simulink model "sim_suspension"  (R2024a)
settings: Solver=ode45  StartTime=0.0  StopTime=3  MaxStep=1e-3  RelTol=1e-3
model workspace (MAT data in the model file):
  road_excitation = 20
undefined symbols (not defined in the file): k, m, r, road_excitation_amplitude, road_excitation_omega, v0, x0
settings Model: Creator=ArrigonDell  LastModifiedBy=Bocchio
settings SolverCC: AlgebraicLoopSolver=TrustRegion
settings DataIOCC: SaveOutput=off  SaveTime=off  ReturnWorkspaceOutputs=off
settings DebuggingCC: UnconnectedInputMsg=warning  UnconnectedOutputMsg=warning  UnconnectedLineMsg=warning  ArithmeticOperatorsInVariantConditions=warning
settings ModelReferenceCC: EnableRefExpFcnMdlSchedulingChecks=on
settings SFSimCC: SimUseLocalCustomCode=off  CustomCodeUndefinedFunction=UseInterfaceOnly
settings RTWCC: RTWUseLocalCustomCode=off  GPUComputeCapability=3.5  DLArmComputeVersion=19.05

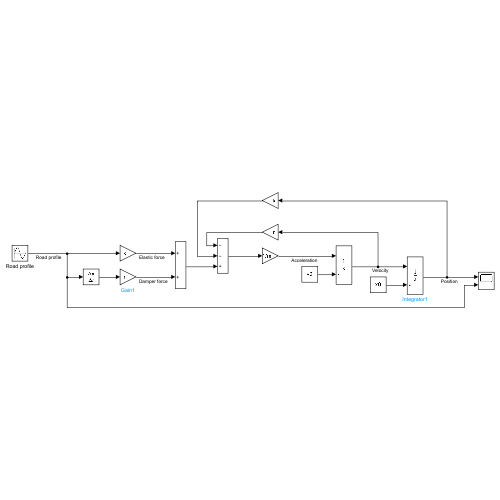
[thumbnail: Simulink's stored preview of the top-level diagram]
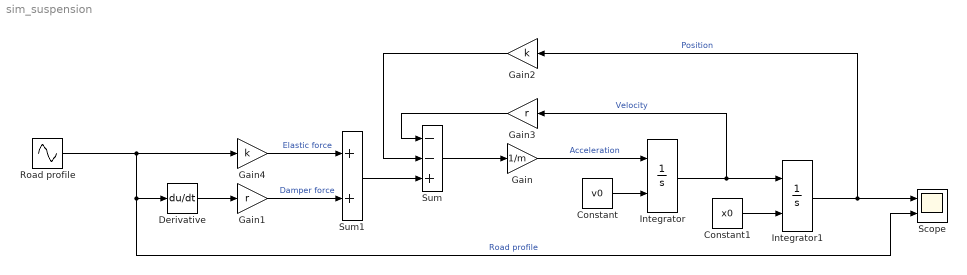
== system sim_suspension ==
  Constant : Constant  Value=v0
  Constant1 : Constant  Value=x0
  Derivative : Derivative
  Gain : Gain  Gain=1/m
  Gain1 : Gain  Gain=r
  Gain2 : Gain  Gain=k
  Gain3 : Gain  Gain=r
  Gain4 : Gain  Gain=k
  Integrator : Integrator  InitialConditionSource=external
  Integrator1 : Integrator  InitialConditionSource=external
  Road profile : Sin  Amplitude=road_excitation_amplitude  Frequency=road_excitation_omega  SampleTime=0
  Scope : Scope  NumInputPorts=2
  Sum : Sum  Inputs=--+
  Sum1 : Sum
  wires:
  Road profile/1 -> Scope/2, Derivative/1, Gain4/1  "Road profile"
  Derivative/1 -> Gain1/1
  Gain3/1 -> Sum/1
  Integrator1/1 -> Gain2/1, Scope/1  "Position"
  Gain4/1 -> Sum1/1  "Elastic force"
  Gain1/1 -> Sum1/2  "Damper force"
  Sum1/1 -> Sum/3
  Gain/1 -> Integrator/1  "Acceleration"
  Sum/1 -> Gain/1
  Constant/1 -> Integrator/2
  Gain2/1 -> Sum/2
  Integrator/1 -> Gain3/1, Integrator1/1  "Velocity"
  Constant1/1 -> Integrator1/2
